simulink model "FOODSLIB"  (Simulink 4.00)
settings: Solver=ode5  SolverMode=SingleTasking  StartTime=0.0  StopTime=0  FixedStep=0  MaxStep=0  RelTol=1e-3  AbsTol=1e-6
undefined symbols (not defined in the file or in its folder): comptype, na, tref, turn
(part 2 of 2)

== system FOODSLIB/Unit  Operations/Single Stage Ultrafiltration/Advanced Transport Level (4) ==
  Hagen-Poiseuille  Model (1) : Subsystem
      settings: RTWFcnNameOpts=Auto  RTWFileNameOpts=Auto
  Mass Transfer (Film Theory) Model (2) : Subsystem
      settings: RTWFcnNameOpts=Auto  RTWFileNameOpts=Auto
  Model Selection : Constant  Value=1
  More Info : Subsystem
      settings: RTWFcnNameOpts=Auto  RTWFileNameOpts=Auto
      mask Display: disp('Help?')
  Mux1 : Mux  Inputs=4
      settings: DisplayOption=none
  Viscosity Model : Constant  Value=6
  out_1 : Outport  Port=1
  wires:
  Mux1/1 -> out_1/1
  Mass Transfer (Film Theory) Model (2)/1(out_1) -> Mux1/4
  Hagen-Poiseuille  Model (1)/1(out_1) -> Mux1/3
  Viscosity Model/1 -> Mux1/1
  Model Selection/1 -> Mux1/2

== system FOODSLIB/Unit  Operations/Single Stage Ultrafiltration/Basic Transport Level (3) ==
  Flux (L/h-m^2) : Constant  Value=17
  out_1 : Outport  Port=1
  wires:
  Flux (L/h-m^2)/1 -> out_1/1

== system FOODSLIB/Unit  Operations/Single Stage Ultrafiltration/Design ==
  Design Level : Constant  Value=4
  Economic Evaluation? : Constant  Value=turn('off')
  Microbial & Quality Assessment? : Constant  Value=turn('off')
  Mux2 : Mux  Inputs=3
      settings: DisplayOption=none
  out_1 : Outport  Port=1
  wires:
  Mux2/1 -> out_1/1
  Design Level/1 -> Mux2/1
  Microbial & Quality Assessment?/1 -> Mux2/2
  Economic Evaluation?/1 -> Mux2/3

== system FOODSLIB/Unit  Operations/Single Stage Ultrafiltration/Mass Balance Level (1) ==
  Ash Rejection Ratio : Constant  Value=[comptype('ash') 0.2]
  Carbohydrate Rejection Ratio : Constant  Value=[comptype('carbohydrate') 0]
  Component Fraction 10 Rejection Ratio : Constant  Value=[0 0]
  Component Fraction 7 Rejection Ratio : Constant  Value=[0 0]
  Component Fraction 8 Rejection Ratio : Constant  Value=[0 0]
  Component Fraction 9 Rejection Ratio : Constant  Value=[0 0]
  Fat Rejection Ratio : Constant  Value=[comptype('fat') 0]
  Fiber Rejection Ratio : Constant  Value=[comptype('fiber') 0]
  Mux : Mux  Inputs=10
      settings: DisplayOption=none
  Protein Rejection Ratio : Constant  Value=[comptype('protein') 0.9]
  Retentate Total Solids (w/w) : Constant  Value=0.2
  out_1 : Outport  Port=1
  wires:
  Fiber Rejection Ratio/1 -> Mux/4
  Carbohydrate Rejection Ratio/1 -> Mux/3
  Fat Rejection Ratio/1 -> Mux/5
  Protein Rejection Ratio/1 -> Mux/2
  Retentate Total Solids (w/w)/1 -> Mux/1
  Mux/1 -> out_1/1
  Ash Rejection Ratio/1 -> Mux/6
  Component Fraction 7 Rejection Ratio/1 -> Mux/7
  Component Fraction 8 Rejection Ratio/1 -> Mux/8
  Component Fraction 9 Rejection Ratio/1 -> Mux/9
  Component Fraction 10 Rejection Ratio/1 -> Mux/10

== system FOODSLIB/Unit  Operations/Single Stage Ultrafiltration/More Info ==
  note: Some Notes
  note: More Notes can go here

== system FOODSLIB/Unit  Operations/Single Stage Ultrafiltration/Ultrafiltration Cost Information ==
  Base Ultrafiltration Costing Model : Subsystem
      settings: RTWFcnNameOpts=Auto  RTWFileNameOpts=Auto
  Equipment Life (y) : Constant  Value=3
  Maintenance Labor (man-h/h operation) : Constant  Value=0.03
  Mux : Mux  Inputs=5
      settings: DisplayOption=none
  Operating Labor (man-h/h operation) : Constant  Value=1
  Salvage Value  (% of initial cost) : Constant  Value=0.1
  out_1 : Outport  Port=1
  wires:
  Maintenance Labor (man-h/h operation)/1 -> Mux/5
  Operating Labor (man-h/h operation)/1 -> Mux/4
  Equipment Life (y)/1 -> Mux/3
  Salvage Value  (% of initial cost)/1 -> Mux/2
  Base Ultrafiltration Costing Model/1(out_1) -> Mux/1
  Mux/1 -> out_1/1

== system FOODSLIB/Unit  Operations/Spray Dryer/Advanced Transport Level (4) ==
  Atomizer - Rotary  Vaned Wheel : Subsystem
      settings: RTWFcnNameOpts=Auto  RTWFileNameOpts=Auto
  Cone Angle (deg. from horizontal) : Constant  Value=60
  Critical  Moisture  Content (wb) : Constant  Value=0.25
  Cylindrical H:D Ratio : Constant  Value=1
  More Info : Subsystem
      settings: RTWFcnNameOpts=Auto  RTWFileNameOpts=Auto
      mask Display: disp('?')
  Mux1 : Mux  Inputs=6
      settings: DisplayOption=none
  Product Density (kg/m^3) : Constant  Value=605
  Viscosity Model : Constant  Value=1
  Out : Outport  Port=1
  wires:
  Mux1/1 -> Out/1
  Atomizer - Rotary  Vaned Wheel/1(out_1) -> Mux1/1
  Critical  Moisture  Content (wb)/1 -> Mux1/2
  Product Density (kg/m^3)/1 -> Mux1/3
  Cylindrical H:D Ratio/1 -> Mux1/4
  Cone Angle (deg. from horizontal)/1 -> Mux1/5
  Viscosity Model/1 -> Mux1/6

== system FOODSLIB/Unit  Operations/Spray Dryer/Design ==
  Design Level : Constant  Value=4
  Economic Evaluation? : Constant  Value=turn('off')
  Microbial & Quality Assessment? : Constant  Value=turn('off')
  Mux2 : Mux  Inputs=3
      settings: DisplayOption=none
  out_1 : Outport  Port=1
  wires:
  Mux2/1 -> out_1/1
  Design Level/1 -> Mux2/1
  Microbial & Quality Assessment?/1 -> Mux2/2
  Economic Evaluation?/1 -> Mux2/3

== system FOODSLIB/Unit  Operations/Spray Dryer/Energy Balance Level (2) ==
  Air Recycle Fraction : Constant  Value=0
  Dryer Air Inlet Temperature (C) : Constant  Value=170
  Dryer Air Outlet Temperature (C) : Constant  Value=90
  Dryer Heat Loss Rate (kJ/h) : Constant  Value=0.0
  Mux : Mux  Inputs=6
      settings: DisplayOption=none
  Operating Pressure (MPa) : Constant  Value=0.101325
  Product Temperature (C) : Constant  Value=75
  Outport : Outport  Port=1
  wires:
  Product Temperature (C)/1 -> Mux/1
  Dryer Air Inlet Temperature (C)/1 -> Mux/2
  Dryer Air Outlet Temperature (C)/1 -> Mux/3
  Mux/1 -> Outport/1
  Operating Pressure (MPa)/1 -> Mux/4
  Air Recycle Fraction/1 -> Mux/6
  Dryer Heat Loss Rate (kJ/h)/1 -> Mux/5

== system FOODSLIB/Unit  Operations/Spray Dryer/Mass Balance Level (1) ==
  Dry Product Total Solids (w/w) : Constant  Value=0.97
  out_1 : Outport  Port=1
  wires:
  Dry Product Total Solids (w/w)/1 -> out_1/1

== system FOODSLIB/Unit  Operations/Spray Dryer/Spray Dryer Cost Information ==
  Base Evaporator Costing Model : Subsystem
      settings: RTWFcnNameOpts=Auto  RTWFileNameOpts=Auto
  Equipment Life (y) : Constant  Value=10
  Maintenance Labor (man-h/h operation) : Constant  Value=0.06
  Mux : Mux  Inputs=5
      settings: DisplayOption=none
  Operating Labor (man-h/h operation) : Constant  Value=1
  Salvage Value  (% of initial cost) : Constant  Value=0.1
  out_1 : Outport  Port=1
  wires:
  Mux/1 -> out_1/1
  Base Evaporator Costing Model/1(out_1) -> Mux/1
  Salvage Value  (% of initial cost)/1 -> Mux/2
  Equipment Life (y)/1 -> Mux/3
  Operating Labor (man-h/h operation)/1 -> Mux/4
  Maintenance Labor (man-h/h operation)/1 -> Mux/5

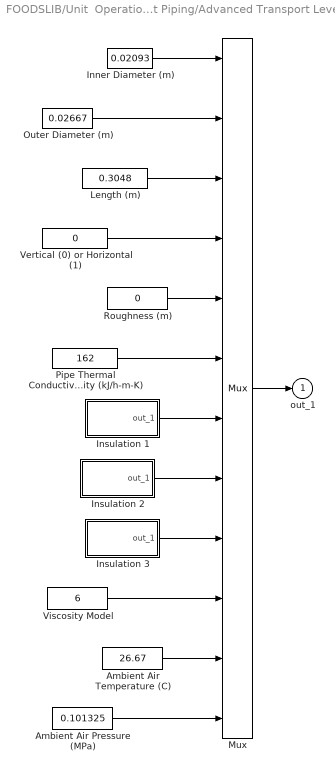
== system FOODSLIB/Unit  Operations/Straight Piping/Advanced Transport Level (4) ==
  Ambient Air Pressure (MPa) : Constant  Value=0.101325
  Ambient Air Temperature (C) : Constant  Value=26.67
  Inner Diameter (m) : Constant  Value=0.02093
  Insulation 1 : Subsystem
      settings: RTWFcnNameOpts=Auto  RTWFileNameOpts=Auto
  Insulation 2 : Subsystem
      settings: RTWFcnNameOpts=Auto  RTWFileNameOpts=Auto
  Insulation 3 : Subsystem
      settings: RTWFcnNameOpts=Auto  RTWFileNameOpts=Auto
  Length (m) : Constant  Value=0.3048
  Mux : Mux  Inputs=12
      settings: DisplayOption=none
  Outer Diameter (m) : Constant  Value=0.02667
  Pipe Thermal Conductivity (kJ/h-m-K) : Constant  Value=162
  Roughness (m) : Constant  Value=0
  Vertical (0) or Horizontal (1) : Constant  Value=0
  Viscosity Model : Constant  Value=6
  out_1 : Outport  Port=1
  wires:
  Inner Diameter (m)/1 -> Mux/1
  Outer Diameter (m)/1 -> Mux/2
  Length (m)/1 -> Mux/3
  Vertical (0) or Horizontal (1)/1 -> Mux/4
  Roughness (m)/1 -> Mux/5
  Pipe Thermal Conductivity (kJ/h-m-K)/1 -> Mux/6
  Insulation 1/1(out_1) -> Mux/7
  Insulation 2/1(out_1) -> Mux/8
  Insulation 3/1(out_1) -> Mux/9
  Mux/1 -> out_1/1
  Viscosity Model/1 -> Mux/10
  Ambient Air Temperature (C)/1 -> Mux/11
  Ambient Air Pressure (MPa)/1 -> Mux/12

== system FOODSLIB/Unit  Operations/Straight Piping/Design ==
  Design Level : Constant  Value=4
  Economic Evaluation? : Constant  Value=turn('off')
  Microbial & Quality Assessment? : Constant  Value=turn('off')
  Mux2 : Mux  Inputs=3
      settings: DisplayOption=none
  out_1 : Outport  Port=1
  wires:
  Mux2/1 -> out_1/1
  Design Level/1 -> Mux2/1
  Microbial & Quality Assessment?/1 -> Mux2/2
  Economic Evaluation?/1 -> Mux2/3

== system FOODSLIB/Unit  Operations/Straight Piping/Pipe Cost Information ==
  Base Evaporator Costing Model : Subsystem
      settings: RTWFcnNameOpts=Auto  RTWFileNameOpts=Auto
  Equipment Life (y) : Constant  Value=3
  Maintenance Labor (man-h/h operation) : Constant  Value=0.03
  Mux : Mux  Inputs=5
      settings: DisplayOption=none
  Operating Labor (man-h/h operation) : Constant  Value=1
  Salvage Value  (% of initial cost) : Constant  Value=0.1
  out_1 : Outport  Port=1
  wires:
  Maintenance Labor (man-h/h operation)/1 -> Mux/5
  Operating Labor (man-h/h operation)/1 -> Mux/4
  Equipment Life (y)/1 -> Mux/3
  Salvage Value  (% of initial cost)/1 -> Mux/2
  Base Evaporator Costing Model/1(out_1) -> Mux/1
  Mux/1 -> out_1/1

== system FOODSLIB/Unit  Operations/Sudden Expansion or Contraction/Advanced Transport Level (4) ==
  Diameter In (m) : Constant  Value=100
  Diameter Out (m) : Constant  Value=0.1023
  Equivalent Straight Pipe Roughness (m) : Constant  Value=0
  Mux : Mux  Inputs=4
      settings: DisplayOption=none
  Viscosity Model : Constant  Value=6
  out_1 : Outport  Port=1
  wires:
  Viscosity Model/1 -> Mux/4
  Equivalent Straight Pipe Roughness (m)/1 -> Mux/3
  Diameter Out (m)/1 -> Mux/2
  Diameter In (m)/1 -> Mux/1
  Mux/1 -> out_1/1

== system FOODSLIB/Unit  Operations/Sudden Expansion or Contraction/Design ==
  Design Level : Constant  Value=4
  Economic Evaluation? : Constant  Value=turn('off')
  Microbial & Quality Assessment? : Constant  Value=turn('off')
  Mux2 : Mux  Inputs=3
      settings: DisplayOption=none
  out_1 : Outport  Port=1
  wires:
  Economic Evaluation?/1 -> Mux2/3
  Microbial & Quality Assessment?/1 -> Mux2/2
  Design Level/1 -> Mux2/1
  Mux2/1 -> out_1/1

== system FOODSLIB/Unit  Operations/Sudden Expansion or Contraction/Fitting Cost Information ==
  Base Evaporator Costing Model : Subsystem
      settings: RTWFcnNameOpts=Auto  RTWFileNameOpts=Auto
  Equipment Life (y) : Constant  Value=3
  Maintenance Labor (man-h/h operation) : Constant  Value=0.03
  Mux : Mux  Inputs=5
      settings: DisplayOption=none
  Operating Labor (man-h/h operation) : Constant  Value=1
  Salvage Value  (% of initial cost) : Constant  Value=0.1
  out_1 : Outport  Port=1
  wires:
  Mux/1 -> out_1/1
  Base Evaporator Costing Model/1(out_1) -> Mux/1
  Salvage Value  (% of initial cost)/1 -> Mux/2
  Equipment Life (y)/1 -> Mux/3
  Operating Labor (man-h/h operation)/1 -> Mux/4
  Maintenance Labor (man-h/h operation)/1 -> Mux/5

== system FOODSLIB/Unit  Operations/Up To 6 Effect  Backward Feed  Evaporator/Advanced Transport Level (4) ==
  Evaporator Model Type (See ?) : Constant  Value=20
  Film Thickness (m) : Constant  Value=.0005
  Initial Guess at Number of Tubes : Constant  Value=35
  Minimum Average Fluid Velocity (m/s) : Constant  Value=2
  More Info : Subsystem
      settings: RTWFcnNameOpts=Auto  RTWFileNameOpts=Auto
      mask Display: disp('?')
  Mux1 : Mux  Inputs=8
      settings: DisplayOption=none
  Pipe Thermal Conductivity  (kJ/h-m-K) : Constant  Value=162
  Pipe Thickness (m) : Constant  Value=0.00391
  Tube Orientation: Horizontal (0); Vertical (1) : Constant  Value=1
  Viscosity Model For Product Side (See ?) : Constant  Value=1
  Out : Outport  Port=1
  wires:
  Mux1/1 -> Out/1
  Evaporator Model Type (See ?)/1 -> Mux1/1
  Tube Orientation: Horizontal (0); Vertical (1)/1 -> Mux1/2
  Viscosity Model For Product Side (See ?)/1 -> Mux1/3
  Pipe Thickness (m)/1 -> Mux1/4
  Pipe Thermal Conductivity  (kJ/h-m-K)/1 -> Mux1/5
  Minimum Average Fluid Velocity (m/s)/1 -> Mux1/6
  Film Thickness (m)/1 -> Mux1/7
  Initial Guess at Number of Tubes/1 -> Mux1/8

== system FOODSLIB/Unit  Operations/Up To 6 Effect  Backward Feed  Evaporator/Basic Transport Level (3) ==
  Effect 1: Overall Heat Transfer Coefficient (kJ/h-m^2-K) : Constant  Value=5400
  Effect 2: Overall Heat Transfer Coefficient (kJ/h-m^2-K) : Constant  Value=3600
  Effect 3: Overall Heat Transfer Coefficient (kJ/h-m^2-K) : Constant  Value=4090
  Effect 4: Overall Heat Transfer Coefficient (kJ/h-m^2-K) : Constant  Value=5400
  Effect 5: Overall Heat Transfer Coefficient (kJ/h-m^2-K) : Constant  Value=5400
  Effect 6: Overall Heat Transfer Coefficient (kJ/h-m^2-K) : Constant  Value=5400
  Inner Pipe Diameter (m) : Constant  Value=0.0525
  Mux1 : Mux  Inputs=8
      settings: DisplayOption=none
  Pipe Length (m) : Constant  Value=2.5
  out_1 : Outport  Port=1
  wires:
  Effect 5: Overall Heat Transfer Coefficient (kJ/h-m^2-K)/1 -> Mux1/5
  Pipe Length (m)/1 -> Mux1/8
  Inner Pipe Diameter (m)/1 -> Mux1/7
  Effect 4: Overall Heat Transfer Coefficient (kJ/h-m^2-K)/1 -> Mux1/4
  Effect 3: Overall Heat Transfer Coefficient (kJ/h-m^2-K)/1 -> Mux1/3
  Effect 2: Overall Heat Transfer Coefficient (kJ/h-m^2-K)/1 -> Mux1/2
  Effect 6: Overall Heat Transfer Coefficient (kJ/h-m^2-K)/1 -> Mux1/6
  Mux1/1 -> out_1/1
  Effect 1: Overall Heat Transfer Coefficient (kJ/h-m^2-K)/1 -> Mux1/1

== system FOODSLIB/Unit  Operations/Up To 6 Effect  Backward Feed  Evaporator/Design ==
  Design Level : Constant  Value=4
  Economic Evaluation? : Constant  Value=turn('off')
  Microbial & Quality Assessment? : Constant  Value=turn('off')
  Mux2 : Mux  Inputs=3
      settings: DisplayOption=none
  out_1 : Outport  Port=1
  wires:
  Mux2/1 -> out_1/1
  Design Level/1 -> Mux2/1
  Microbial & Quality Assessment?/1 -> Mux2/2
  Economic Evaluation?/1 -> Mux2/3

== system FOODSLIB/Unit  Operations/Up To 6 Effect  Backward Feed  Evaporator/Energy Balance Level (2) ==
  Boiling Point Rise Model : Constant  Value=3
  Exit Steam Quality : Constant  Value=0
  Last Effect Operating Pressure (MPa) : Constant  Value=0.007
  More Info : Subsystem
      settings: RTWFcnNameOpts=Auto  RTWFileNameOpts=Auto
      mask Display: disp('?')
  Mux : Mux  Inputs=3
      settings: DisplayOption=none
  out_1 : Outport  Port=1
  wires:
  Exit Steam Quality/1 -> Mux/2
  Last Effect Operating Pressure (MPa)/1 -> Mux/1
  Mux/1 -> out_1/1
  Boiling Point Rise Model/1 -> Mux/3

== system FOODSLIB/Unit  Operations/Up To 6 Effect  Backward Feed  Evaporator/Evaporator Cost Information ==
  Base Evaporator Costing Model : Subsystem
      settings: RTWFcnNameOpts=Auto  RTWFileNameOpts=Auto
  Equipment Life (y) : Constant  Value=10
  Maintenance Labor (man-h/h operation) : Constant  Value=0.015
  Mux : Mux  Inputs=5
      settings: DisplayOption=none
  Operating Labor (man-h/h operation) : Constant  Value=0.25
  Salvage Value  (% of initial cost) : Constant  Value=0.1
  out_1 : Outport  Port=1
  wires:
  Maintenance Labor (man-h/h operation)/1 -> Mux/5
  Operating Labor (man-h/h operation)/1 -> Mux/4
  Equipment Life (y)/1 -> Mux/3
  Salvage Value  (% of initial cost)/1 -> Mux/2
  Base Evaporator Costing Model/1(out_1) -> Mux/1
  Mux/1 -> out_1/1

== system FOODSLIB/Unit  Operations/Up To 6 Effect  Backward Feed  Evaporator/Mass Balance Level (1) ==
  Mux : Mux  Inputs=2
      settings: DisplayOption=none
  Number of Effects (Limited to 6) : Constant  Value=3
  Total Solids of Liquid Concentrate (w/w) : Constant  Value=0.48
  out_1 : Outport  Port=1
  wires:
  Total Solids of Liquid Concentrate (w/w)/1 -> Mux/2
  Number of Effects (Limited to 6)/1 -> Mux/1
  Mux/1 -> out_1/1

== system FOODSLIB/Unit  Operations/Up To 6 Effect  Forward Feed  Evaporator/Advanced Transport Level (4) ==
  Evaporator Model Type (See ?) : Constant  Value=20
  Film Thickness (m) : Constant  Value=.0005
  Initial Guess at Number of Tubes : Constant  Value=35
  Minimum Average Fluid Velocity (m/s) : Constant  Value=2
  More Info : Subsystem
      settings: RTWFcnNameOpts=Auto  RTWFileNameOpts=Auto
      mask Display: disp('?')
  Mux1 : Mux  Inputs=8
      settings: DisplayOption=none
  Pipe Thermal Conductivity  (kJ/h-m-K) : Constant  Value=162
  Pipe Thickness (m) : Constant  Value=0.00391
  Tube Orientation: Horizontal (0); Vertical (1) : Constant  Value=1
  Viscosity Model For Product Side (See ?) : Constant  Value=1
  Out : Outport  Port=1
  wires:
  Mux1/1 -> Out/1
  Evaporator Model Type (See ?)/1 -> Mux1/1
  Tube Orientation: Horizontal (0); Vertical (1)/1 -> Mux1/2
  Viscosity Model For Product Side (See ?)/1 -> Mux1/3
  Pipe Thickness (m)/1 -> Mux1/4
  Pipe Thermal Conductivity  (kJ/h-m-K)/1 -> Mux1/5
  Minimum Average Fluid Velocity (m/s)/1 -> Mux1/6
  Film Thickness (m)/1 -> Mux1/7
  Initial Guess at Number of Tubes/1 -> Mux1/8

== system FOODSLIB/Unit  Operations/Up To 6 Effect  Forward Feed  Evaporator/Basic Transport Level (3) ==
  Effect 1: Overall Heat Transfer Coefficient (kJ/h-m^2-K) : Constant  Value=5400
  Effect 2: Overall Heat Transfer Coefficient (kJ/h-m^2-K) : Constant  Value=3600
  Effect 3: Overall Heat Transfer Coefficient (kJ/h-m^2-K) : Constant  Value=4090
  Effect 4: Overall Heat Transfer Coefficient (kJ/h-m^2-K) : Constant  Value=5400
  Effect 5: Overall Heat Transfer Coefficient (kJ/h-m^2-K) : Constant  Value=5400
  Effect 6: Overall Heat Transfer Coefficient (kJ/h-m^2-K) : Constant  Value=5400
  Inner Pipe Diameter (m) : Constant  Value=0.0525
  Mux1 : Mux  Inputs=8
      settings: DisplayOption=none
  Pipe Length (m) : Constant  Value=2.5
  out_1 : Outport  Port=1
  wires:
  Effect 5: Overall Heat Transfer Coefficient (kJ/h-m^2-K)/1 -> Mux1/5
  Pipe Length (m)/1 -> Mux1/8
  Inner Pipe Diameter (m)/1 -> Mux1/7
  Effect 4: Overall Heat Transfer Coefficient (kJ/h-m^2-K)/1 -> Mux1/4
  Effect 3: Overall Heat Transfer Coefficient (kJ/h-m^2-K)/1 -> Mux1/3
  Effect 2: Overall Heat Transfer Coefficient (kJ/h-m^2-K)/1 -> Mux1/2
  Effect 6: Overall Heat Transfer Coefficient (kJ/h-m^2-K)/1 -> Mux1/6
  Mux1/1 -> out_1/1
  Effect 1: Overall Heat Transfer Coefficient (kJ/h-m^2-K)/1 -> Mux1/1

== system FOODSLIB/Unit  Operations/Up To 6 Effect  Forward Feed  Evaporator/Design ==
  Design Level : Constant  Value=4
  Economic Evaluation? : Constant  Value=turn('off')
  Microbial & Quality Assessment? : Constant  Value=turn('off')
  Mux2 : Mux  Inputs=3
      settings: DisplayOption=none
  out_1 : Outport  Port=1
  wires:
  Mux2/1 -> out_1/1
  Design Level/1 -> Mux2/1
  Microbial & Quality Assessment?/1 -> Mux2/2
  Economic Evaluation?/1 -> Mux2/3

== system FOODSLIB/Unit  Operations/Up To 6 Effect  Forward Feed  Evaporator/Energy Balance Level (2) ==
  Boiling Point Rise Model : Constant  Value=3
  Exit Steam Quality : Constant  Value=0
  Last Effect Operating Pressure (MPa) : Constant  Value=0.007
  More Info : Subsystem
      settings: RTWFcnNameOpts=Auto  RTWFileNameOpts=Auto
      mask Display: disp('?')
  Mux : Mux  Inputs=3
      settings: DisplayOption=none
  out_1 : Outport  Port=1
  wires:
  Exit Steam Quality/1 -> Mux/2
  Last Effect Operating Pressure (MPa)/1 -> Mux/1
  Mux/1 -> out_1/1
  Boiling Point Rise Model/1 -> Mux/3

== system FOODSLIB/Unit  Operations/Up To 6 Effect  Forward Feed  Evaporator/Evaporator Cost Information ==
  Base Evaporator Costing Model : Subsystem
      settings: RTWFcnNameOpts=Auto  RTWFileNameOpts=Auto
  Equipment Life (y) : Constant  Value=10
  Maintenance Labor (man-h/h operation) : Constant  Value=0.015
  Mux : Mux  Inputs=5
      settings: DisplayOption=none
  Operating Labor (man-h/h operation) : Constant  Value=0.25
  Salvage Value  (% of initial cost) : Constant  Value=0.1
  out_1 : Outport  Port=1
  wires:
  Maintenance Labor (man-h/h operation)/1 -> Mux/5
  Operating Labor (man-h/h operation)/1 -> Mux/4
  Equipment Life (y)/1 -> Mux/3
  Salvage Value  (% of initial cost)/1 -> Mux/2
  Base Evaporator Costing Model/1(out_1) -> Mux/1
  Mux/1 -> out_1/1

== system FOODSLIB/Unit  Operations/Up To 6 Effect  Forward Feed  Evaporator/Mass Balance Level (1) ==
  Mux : Mux  Inputs=2
      settings: DisplayOption=none
  Number of Effects (Limited to 6) : Constant  Value=3
  Total Solids of Liquid Concentrate (w/w) : Constant  Value=0.48
  out_1 : Outport  Port=1
  wires:
  Total Solids of Liquid Concentrate (w/w)/1 -> Mux/2
  Number of Effects (Limited to 6)/1 -> Mux/1
  Mux/1 -> out_1/1

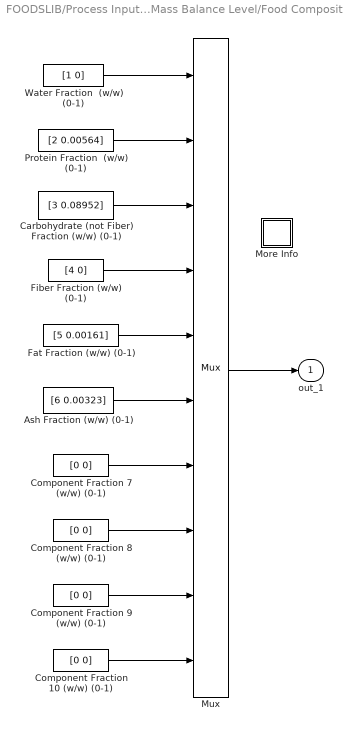
== system FOODSLIB/Process Inputs/Food/Mass Balance Level/Food Composition ==
  Ash Fraction (w/w) (0-1) : Constant  Value=[6 0.00323]
  Carbohydrate (not Fiber) Fraction (w/w) (0-1) : Constant  Value=[3 0.08952]
  Component Fraction 10 (w/w) (0-1) : Constant  Value=[0 0]
  Component Fraction 7 (w/w) (0-1) : Constant  Value=[0 0]
  Component Fraction 8 (w/w) (0-1) : Constant  Value=[0 0]
  Component Fraction 9 (w/w) (0-1) : Constant  Value=[0 0]
  Fat Fraction (w/w) (0-1) : Constant  Value=[5 0.00161]
  Fiber Fraction (w/w) (0-1) : Constant  Value=[4 0]
  More Info : Subsystem
      settings: RTWFcnNameOpts=Auto  RTWFileNameOpts=Auto
      mask Display: disp('?')
  Mux : Mux  Inputs=10
      settings: DisplayOption=none
  Protein Fraction  (w/w) (0-1) : Constant  Value=[2 0.00564]
  Water Fraction  (w/w) (0-1) : Constant  Value=[1 0]
  out_1 : Outport  Port=1
  wires:
  Mux/1 -> out_1/1
  Protein Fraction  (w/w) (0-1)/1 -> Mux/2
  Carbohydrate (not Fiber) Fraction (w/w) (0-1)/1 -> Mux/3
  Water Fraction  (w/w) (0-1)/1 -> Mux/1
  Fiber Fraction (w/w) (0-1)/1 -> Mux/4
  Fat Fraction (w/w) (0-1)/1 -> Mux/5
  Ash Fraction (w/w) (0-1)/1 -> Mux/6
  Component Fraction 7 (w/w) (0-1)/1 -> Mux/7
  Component Fraction 8 (w/w) (0-1)/1 -> Mux/8
  Component Fraction 9 (w/w) (0-1)/1 -> Mux/9
  Component Fraction 10 (w/w) (0-1)/1 -> Mux/10

== system FOODSLIB/Process Inputs/Steam Source/Economics Level/More Info ==
  note: Steam Source Costs are currently NOT set in this block.
      | Rather, they are set within ECONANAL.
      | (na = not available = 0)

== system FOODSLIB/Process Inputs/Steam Source/Energy Balance Level/More Info ==
  note: SUPER-HEATED STATE: Both the Temperature and Pressure must be set.
      | The Quality should be set to a value of 2.
  note: VAPOR-LIQUID STATE: Either the Temperature OR the Pressure may be set.
      | If both properties are set, the pressure will be used to determine the saturated
      | temperature. The saturated temperature will be used throughout the model.

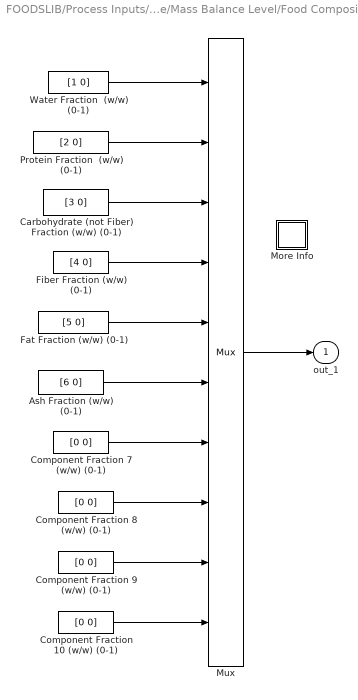
== system FOODSLIB/Process Inputs/Steam w/ known Mass Flowrate/Mass Balance Level/Food Composition ==
  Ash Fraction (w/w) (0-1) : Constant  Value=[6 0]
  Carbohydrate (not Fiber) Fraction (w/w) (0-1) : Constant  Value=[3 0]
  Component Fraction 10 (w/w) (0-1) : Constant  Value=[0 0]
  Component Fraction 7 (w/w) (0-1) : Constant  Value=[0 0]
  Component Fraction 8 (w/w) (0-1) : Constant  Value=[0 0]
  Component Fraction 9 (w/w) (0-1) : Constant  Value=[0 0]
  Fat Fraction (w/w) (0-1) : Constant  Value=[5 0]
  Fiber Fraction (w/w) (0-1) : Constant  Value=[4 0]
  More Info : Subsystem
      settings: RTWFcnNameOpts=Auto  RTWFileNameOpts=Auto
      mask Display: disp('?')
  Mux : Mux  Inputs=10
      settings: DisplayOption=none
  Protein Fraction  (w/w) (0-1) : Constant  Value=[2 0]
  Water Fraction  (w/w) (0-1) : Constant  Value=[1 0]
  out_1 : Outport  Port=1
  wires:
  Component Fraction 10 (w/w) (0-1)/1 -> Mux/10
  Component Fraction 9 (w/w) (0-1)/1 -> Mux/9
  Component Fraction 8 (w/w) (0-1)/1 -> Mux/8
  Component Fraction 7 (w/w) (0-1)/1 -> Mux/7
  Ash Fraction (w/w) (0-1)/1 -> Mux/6
  Fat Fraction (w/w) (0-1)/1 -> Mux/5
  Fiber Fraction (w/w) (0-1)/1 -> Mux/4
  Water Fraction  (w/w) (0-1)/1 -> Mux/1
  Carbohydrate (not Fiber) Fraction (w/w) (0-1)/1 -> Mux/3
  Protein Fraction  (w/w) (0-1)/1 -> Mux/2
  Mux/1 -> out_1/1

== system FOODSLIB/Process Inputs/Water Source/Economics Level/More Info ==
  note: Water Source Costs are currently NOT set in this block.
      | Rather, they are set within ECONANAL.
      | (na = not available = 0)

== system FOODSLIB/Process Inputs/Water Source/Energy Balance Level/More Info ==
  note: To specifiy a water source, the Quality must be set to zero.
  note: Only the Temperature may be set.

== system FOODSLIB/Unit  Operations/Heat Exchanger/Energy Balance Level (2)/More Info ==
  note: Flow Configuration:
      | Co-Current = 0
      | Counter-Current = 1

== system FOODSLIB/Unit  Operations/Heat Exchanger/Heat Exchanger Cost Information/Base Heat Exchanger Costing Model ==
  Base Cost ($) : Constant  Value=5500
  Base MSI : Constant  Value=300
  Base Size (m^2) : Constant  Value=13.9
  Maximum Size (m^2) : Constant  Value=18.6
  Minimim Size (m^2) : Constant  Value=9.3
  Mux : Mux  Inputs=6
      settings: DisplayOption=none
  Scaling Index : Constant  Value=0.65
  out_1 : Outport  Port=1
  wires:
  Maximum Size (m^2)/1 -> Mux/6
  Minimim Size (m^2)/1 -> Mux/5
  Scaling Index/1 -> Mux/4
  Base Cost ($)/1 -> Mux/3
  Base Size (m^2)/1 -> Mux/2
  Base MSI/1 -> Mux/1
  Mux/1 -> out_1/1

== system FOODSLIB/Unit  Operations/Holding Tube/Holding Tube Cost Information/Base Evaporator Costing Model ==
  Base Cost ($/m) : Constant  Value=164
  Base MSI : Constant  Value=904
  Base Size: Nominal Diameter (m) : Constant  Value=0.1016
  Maximum Size: Nominal Diameter (m) : Constant  Value=0.680
  Minimim Size:  Nominal Diameter (m) : Constant  Value=0.0178
  Mux : Mux  Inputs=6
      settings: DisplayOption=none
  Scaling Index : Constant  Value=0.973
  out_1 : Outport  Port=1
  wires:
  Mux/1 -> out_1/1
  Base MSI/1 -> Mux/1
  Base Size: Nominal Diameter (m)/1 -> Mux/2
  Base Cost ($/m)/1 -> Mux/3
  Scaling Index/1 -> Mux/4
  Minimim Size:  Nominal Diameter (m)/1 -> Mux/5
  Maximum Size: Nominal Diameter (m)/1 -> Mux/6

== system FOODSLIB/Unit  Operations/Mass Split/Evaporator Cost Information/Base Mass Split Costing Model ==
  Base Cost ($) : Constant  Value=110150
  Base MSI : Constant  Value=904
  Base Size : Constant  Value=1
  Maximum Size : Constant  Value=1
  Minimim Size : Constant  Value=1
  Mux : Mux  Inputs=6
      settings: DisplayOption=none
  Scaling Index : Constant  Value=0.54
  out_1 : Outport  Port=1
  wires:
  Maximum Size/1 -> Mux/6
  Minimim Size/1 -> Mux/5
  Scaling Index/1 -> Mux/4
  Base Cost ($)/1 -> Mux/3
  Base Size/1 -> Mux/2
  Base MSI/1 -> Mux/1
  Mux/1 -> out_1/1

== system FOODSLIB/Unit  Operations/Pipe Fitting/Fitting Cost Information/Base Evaporator Costing Model ==
  Base Cost ($) : Constant  Value=110150
  Base MSI : Constant  Value=904
  Base Size (m^2) : Constant  Value=100
  Maximum Size (m^2) : Constant  Value=740
  Minimim Size (m^2) : Constant  Value=9.3
  Mux : Mux  Inputs=6
      settings: DisplayOption=none
  Scaling Index : Constant  Value=0.54
  out_1 : Outport  Port=1
  wires:
  Mux/1 -> out_1/1
  Base MSI/1 -> Mux/1
  Base Size (m^2)/1 -> Mux/2
  Base Cost ($)/1 -> Mux/3
  Scaling Index/1 -> Mux/4
  Minimim Size (m^2)/1 -> Mux/5
  Maximum Size (m^2)/1 -> Mux/6

== system FOODSLIB/Unit  Operations/Point Mix/Point Mix Cost Information/Base Mass Split Costing Model ==
  Base Cost ($) : Constant  Value=110150
  Base MSI : Constant  Value=904
  Base Size : Constant  Value=1
  Maximum Size : Constant  Value=1
  Minimim Size : Constant  Value=1
  Mux : Mux  Inputs=6
      settings: DisplayOption=none
  Scaling Index : Constant  Value=0.54
  out_1 : Outport  Port=1
  wires:
  Maximum Size/1 -> Mux/6
  Minimim Size/1 -> Mux/5
  Scaling Index/1 -> Mux/4
  Base Cost ($)/1 -> Mux/3
  Base Size/1 -> Mux/2
  Base MSI/1 -> Mux/1
  Mux/1 -> out_1/1

== system FOODSLIB/Unit  Operations/Point Mix 3/Point Mix Cost Information/Base Mass Split Costing Model ==
  Base Cost ($) : Constant  Value=110150
  Base MSI : Constant  Value=904
  Base Size : Constant  Value=1
  Maximum Size : Constant  Value=1
  Minimim Size : Constant  Value=1
  Mux : Mux  Inputs=6
      settings: DisplayOption=none
  Scaling Index : Constant  Value=0.54
  out_1 : Outport  Port=1
  wires:
  Mux/1 -> out_1/1
  Base MSI/1 -> Mux/1
  Base Size/1 -> Mux/2
  Base Cost ($)/1 -> Mux/3
  Scaling Index/1 -> Mux/4
  Minimim Size/1 -> Mux/5
  Maximum Size/1 -> Mux/6

== system FOODSLIB/Unit  Operations/Pump/Pump Cost Information/Base Evaporator Costing Model ==
  Base Cost ($) : Constant  Value=110150
  Base MSI : Constant  Value=904
  Base Size: Nominal Diameter (m) : Constant  Value=0.0254
  Maximum Size: Nominal Diameter (m) : Constant  Value=0.03
  Minimim Size:  Nominal Diameter (m) : Constant  Value=0.01
  Mux : Mux  Inputs=6
      settings: DisplayOption=none
  Scaling Index : Constant  Value=0.54
  out_1 : Outport  Port=1
  wires:
  Mux/1 -> out_1/1
  Base MSI/1 -> Mux/1
  Base Size: Nominal Diameter (m)/1 -> Mux/2
  Base Cost ($)/1 -> Mux/3
  Scaling Index/1 -> Mux/4
  Minimim Size:  Nominal Diameter (m)/1 -> Mux/5
  Maximum Size: Nominal Diameter (m)/1 -> Mux/6

== system FOODSLIB/Unit  Operations/Single Effect Evaporator/Advanced Transport Level (4)/More Info ==
  note: Evaporator Model Types currently include:
      | Vertical-tube recirulating evaporator - natural circulation = 1
      | Vertical-tube recirculation evaporator - forced circulation = 2

== system FOODSLIB/Unit  Operations/Single Effect Evaporator/Energy Balance Level (2)/More Info ==
  note: Boiling Point Rise Models currently include:
      | None = 0
      | Molecular Concentration = 1
      | Sugar Solutions = 2

== system FOODSLIB/Unit  Operations/Single Effect Evaporator/Evaporator Cost Information/Base Evaporator Costing Model ==
  Base Cost ($) : Constant  Value=23000
  Base MSI : Constant  Value=300
  Base Size (m^2) : Constant  Value=92.9
  Maximum Size (m^2) : Constant  Value=9290.3
  Minimim Size (m^2) : Constant  Value=0.93
  Mux : Mux  Inputs=6
      settings: DisplayOption=none
  Scaling Index : Constant  Value=0.68
  out_1 : Outport  Port=1
  wires:
  Mux/1 -> out_1/1
  Maximum Size (m^2)/1 -> Mux/6
  Minimim Size (m^2)/1 -> Mux/5
  Scaling Index/1 -> Mux/4
  Base Cost ($)/1 -> Mux/3
  Base Size (m^2)/1 -> Mux/2
  Base MSI/1 -> Mux/1

== system FOODSLIB/Unit  Operations/Single Stage Ultrafiltration/Advanced Transport Level (4)/Hagen-Poiseuille  Model (1) ==
  Mean Pore Diameter (microns) : Constant  Value=0.0175
  Mux : Mux  Inputs=4
      settings: DisplayOption=none
  Pore Density (pores/cm^2) : Constant  Value=3e9
  Skin thickness (microns) : Constant  Value=0.2
  Transmembrane Pressure (MPa) : Constant  Value=0.1
  out_1 : Outport  Port=1
  wires:
  Pore Density (pores/cm^2)/1 -> Mux/4
  Skin thickness (microns)/1 -> Mux/3
  Mean Pore Diameter (microns)/1 -> Mux/2
  Transmembrane Pressure (MPa)/1 -> Mux/1
  Mux/1 -> out_1/1

== system FOODSLIB/Unit  Operations/Single Stage Ultrafiltration/Advanced Transport Level (4)/Mass Transfer (Film Theory) Model (2) ==
  Diffusivity (cm^2/s) : Constant  Value=7e-7
  Gel layer concentration (w/w) : Constant  Value=0.22
  Hydraulic (tube/fiber) Diameter (m) : Constant  Value=0.0011
  Model Constants : Subsystem
      settings: RTWFcnNameOpts=Auto  RTWFileNameOpts=Auto
  Mux : Mux  Inputs=6
      settings: DisplayOption=none
  Number of tubes/fibers : Constant  Value=660
  Tube/Fiber Length (m) : Constant  Value=0.635
  out_1 : Outport  Port=1
  wires:
  Gel layer concentration (w/w)/1 -> Mux/5
  Model Constants/1(out_1) -> Mux/6
  Diffusivity (cm^2/s)/1 -> Mux/4
  Number of tubes/fibers/1 -> Mux/3
  Tube/Fiber Length (m)/1 -> Mux/2
  Hydraulic (tube/fiber) Diameter (m)/1 -> Mux/1
  Mux/1 -> out_1/1

== system FOODSLIB/Unit  Operations/Single Stage Ultrafiltration/Advanced Transport Level (4)/More Info ==
  note: Evaporator Model Types currently include:
      | Vertical-tube recirulating evaporator - natural circulation = 1
      | Vertical-tube recirculation evaporator - forced circulation = 2

== system FOODSLIB/Unit  Operations/Single Stage Ultrafiltration/Ultrafiltration Cost Information/Base Ultrafiltration Costing Model ==
  Base Cost ($) : Constant  Value=110150
  Base MSI : Constant  Value=904
  Base Size (m^2) : Constant  Value=100
  Maximum Size (m^2) : Constant  Value=740
  Minimim Size (m^2) : Constant  Value=9.3
  Mux : Mux  Inputs=6
      settings: DisplayOption=none
  Scaling Index : Constant  Value=0.54
  out_1 : Outport  Port=1
  wires:
  Maximum Size (m^2)/1 -> Mux/6
  Minimim Size (m^2)/1 -> Mux/5
  Scaling Index/1 -> Mux/4
  Base Cost ($)/1 -> Mux/3
  Base Size (m^2)/1 -> Mux/2
  Base MSI/1 -> Mux/1
  Mux/1 -> out_1/1

== system FOODSLIB/Unit  Operations/Spray Dryer/Advanced Transport Level (4)/Atomizer - Rotary  Vaned Wheel ==
  "Mean Droplet Diameter (m) {Value overrides calculated value}" : Constant  Value=0
  Mux : Mux  Inputs=5
      settings: DisplayOption=none
  Number of Vanes : Constant  Value=36
  Vane Height (m) : Constant  Value=0.03
  Wheel Diameter (m) : Constant  Value=0.25
  Wheel Speed (rpm) : Constant  Value=12000
  out_1 : Outport  Port=1
  wires:
  Vane Height (m)/1 -> Mux/5
  Number of Vanes/1 -> Mux/4
  Wheel Diameter (m)/1 -> Mux/3
  Wheel Speed (rpm)/1 -> Mux/2
  "Mean Droplet Diameter (m) {Value overrides calculated value}"/1 -> Mux/1
  Mux/1 -> out_1/1

== system FOODSLIB/Unit  Operations/Spray Dryer/Advanced Transport Level (4)/More Info ==
  note: Evaporator Model Types currently include:
      | Vertical-tube recirulating evaporator - natural circulation = 1
      | Vertical-tube recirculation evaporator - forced circulation = 2

== system FOODSLIB/Unit  Operations/Spray Dryer/Spray Dryer Cost Information/Base Evaporator Costing Model ==
  Base Cost ($) : Constant  Value=150000
  Base MSI : Constant  Value=300
  Base Size (kg water/h) : Constant  Value=2268.
  Maximum Size (kg water/h) : Constant  Value=9071.8
  Minimim Size (kg water/h) : Constant  Value=113.4
  Mux : Mux  Inputs=6
      settings: DisplayOption=none
  Scaling Index : Constant  Value=0.71
  out_1 : Outport  Port=1
  wires:
  Mux/1 -> out_1/1
  Base MSI/1 -> Mux/1
  Base Size (kg water/h)/1 -> Mux/2
  Base Cost ($)/1 -> Mux/3
  Scaling Index/1 -> Mux/4
  Minimim Size (kg water/h)/1 -> Mux/5
  Maximum Size (kg water/h)/1 -> Mux/6

== system FOODSLIB/Unit  Operations/Straight Piping/Advanced Transport Level (4)/Insulation 1 ==
  Mux1 : Mux  Inputs=2
      settings: DisplayOption=none
  Thermal Conductivity (kJ/h-m-K) : Constant  Value=0.2304
  Thickness (m) : Constant  Value=0.0381
  out_1 : Outport  Port=1
  wires:
  Mux1/1 -> out_1/1
  Thickness (m)/1 -> Mux1/1
  Thermal Conductivity (kJ/h-m-K)/1 -> Mux1/2

== system FOODSLIB/Unit  Operations/Straight Piping/Advanced Transport Level (4)/Insulation 2 ==
  Mux1 : Mux  Inputs=2
      settings: DisplayOption=none
  Thermal Conductivity (kJ/h-m-K) : Constant  Value=0.0
  Thickness (m) : Constant  Value=0.0
  out_1 : Outport  Port=1
  wires:
  Mux1/1 -> out_1/1
  Thickness (m)/1 -> Mux1/1
  Thermal Conductivity (kJ/h-m-K)/1 -> Mux1/2

== system FOODSLIB/Unit  Operations/Straight Piping/Advanced Transport Level (4)/Insulation 3 ==
  Mux1 : Mux  Inputs=2
      settings: DisplayOption=none
  Thermal Conductivity (kJ/h-m-K) : Constant  Value=0.0
  Thickness (m) : Constant  Value=0
  out_1 : Outport  Port=1
  wires:
  Mux1/1 -> out_1/1
  Thickness (m)/1 -> Mux1/1
  Thermal Conductivity (kJ/h-m-K)/1 -> Mux1/2

== system FOODSLIB/Unit  Operations/Straight Piping/Pipe Cost Information/Base Evaporator Costing Model ==
  Base Cost ($) : Constant  Value=110150
  Base MSI : Constant  Value=904
  Base Size: Nominal Diameter (m) : Constant  Value=0.0254
  Maximum Size: Nominal Diameter (m) : Constant  Value=0.03
  Minimim Size:  Nominal Diameter (m) : Constant  Value=0.01
  Mux : Mux  Inputs=6
      settings: DisplayOption=none
  Scaling Index : Constant  Value=0.54
  out_1 : Outport  Port=1
  wires:
  Maximum Size: Nominal Diameter (m)/1 -> Mux/6
  Minimim Size:  Nominal Diameter (m)/1 -> Mux/5
  Scaling Index/1 -> Mux/4
  Base Cost ($)/1 -> Mux/3
  Base Size: Nominal Diameter (m)/1 -> Mux/2
  Base MSI/1 -> Mux/1
  Mux/1 -> out_1/1

== system FOODSLIB/Unit  Operations/Sudden Expansion or Contraction/Fitting Cost Information/Base Evaporator Costing Model ==
  Base Cost ($) : Constant  Value=110150
  Base MSI : Constant  Value=904
  Base Size (m^2) : Constant  Value=100
  Maximum Size (m^2) : Constant  Value=740
  Minimim Size (m^2) : Constant  Value=9.3
  Mux : Mux  Inputs=6
      settings: DisplayOption=none
  Scaling Index : Constant  Value=0.54
  out_1 : Outport  Port=1
  wires:
  Mux/1 -> out_1/1
  Base MSI/1 -> Mux/1
  Base Size (m^2)/1 -> Mux/2
  Base Cost ($)/1 -> Mux/3
  Scaling Index/1 -> Mux/4
  Minimim Size (m^2)/1 -> Mux/5
  Maximum Size (m^2)/1 -> Mux/6

== system FOODSLIB/Unit  Operations/Up To 6 Effect  Backward Feed  Evaporator/Advanced Transport Level (4)/More Info ==
  note: Evaporator Model Types currently include:
      | Vertical-tube recirulating evaporator - natural circulation = 1
      | Vertical-tube recirculation evaporator - forced circulation = 2

== system FOODSLIB/Unit  Operations/Up To 6 Effect  Backward Feed  Evaporator/Energy Balance Level (2)/More Info ==
  note: Boiling Point Rise Models currently include:
      | None = 0
      | Molecular Concentration = 1
      | Sugar Solutions = 2

== system FOODSLIB/Unit  Operations/Up To 6 Effect  Backward Feed  Evaporator/Evaporator Cost Information/Base Evaporator Costing Model ==
  Base Cost ($) : Constant  Value=23000
  Base MSI : Constant  Value=300
  Base Size (m^2) : Constant  Value=92.9
  Maximum Size (m^2) : Constant  Value=9290.3
  Minimim Size (m^2) : Constant  Value=0.93
  Mux : Mux  Inputs=6
      settings: DisplayOption=none
  Scaling Index : Constant  Value=0.68
  out_1 : Outport  Port=1
  wires:
  Maximum Size (m^2)/1 -> Mux/6
  Minimim Size (m^2)/1 -> Mux/5
  Scaling Index/1 -> Mux/4
  Base Cost ($)/1 -> Mux/3
  Base Size (m^2)/1 -> Mux/2
  Base MSI/1 -> Mux/1
  Mux/1 -> out_1/1

== system FOODSLIB/Unit  Operations/Up To 6 Effect  Forward Feed  Evaporator/Advanced Transport Level (4)/More Info ==
  note: Evaporator Model Types currently include:
      | Vertical-tube recirulating evaporator - natural circulation = 1
      | Vertical-tube recirculation evaporator - forced circulation = 2

== system FOODSLIB/Unit  Operations/Up To 6 Effect  Forward Feed  Evaporator/Energy Balance Level (2)/More Info ==
  note: Boiling Point Rise Models currently include:
      | None = 0
      | Molecular Concentration = 1
      | Sugar Solutions = 2

== system FOODSLIB/Unit  Operations/Up To 6 Effect  Forward Feed  Evaporator/Evaporator Cost Information/Base Evaporator Costing Model ==
  Base Cost ($) : Constant  Value=23000
  Base MSI : Constant  Value=300
  Base Size (m^2) : Constant  Value=92.9
  Maximum Size (m^2) : Constant  Value=9290.3
  Minimim Size (m^2) : Constant  Value=0.93
  Mux : Mux  Inputs=6
      settings: DisplayOption=none
  Scaling Index : Constant  Value=0.68
  out_1 : Outport  Port=1
  wires:
  Maximum Size (m^2)/1 -> Mux/6
  Minimim Size (m^2)/1 -> Mux/5
  Scaling Index/1 -> Mux/4
  Base Cost ($)/1 -> Mux/3
  Base Size (m^2)/1 -> Mux/2
  Base MSI/1 -> Mux/1
  Mux/1 -> out_1/1

== system FOODSLIB/Process Inputs/Food/Mass Balance Level/Food Composition/More Info ==
  note: Food Stream Compositions may be specified with up to 10 components.
      | The first component must ALWAYS be water.
  note: A check is made by the S-function feeds.m to ensure that the mass fractions
      | sum to 1. In the event that the sum of the mass fractions is less than 1,
      | the watermass fraction is recalculated to bring the sum up to 1.
  note: Each component is described by two values: type and mass fraction.
      | The values must be entered as [type mass_fraction] in the Constant Block.
      |
      | Example: A protein concentration of 4% (w/w) is entered as [2 0.04]
  note: Currently recognized component types are:
      | water =1
      | protein = 2
      | carbohydrate (not fiber) = 3
      | fiber = 4
      | fat = 5
      | ash = 6

== system FOODSLIB/Process Inputs/Steam w/ known Mass Flowrate/Mass Balance Level/Food Composition/More Info ==
  note: Currently recognized component types are:
      | water =1
      | protein = 2
      | carbohydrate (not fiber) = 3
      | fiber = 4
      | fat = 5
      | ash = 6
  note: Each component is described by two values: type and mass fraction.
      | The values must be entered as [type mass_fraction] in the Constant Block.
  note: A check is made by feeds.m to ensure that the mass fractions sum to 1.
      | In the event that the sum of the mass fractions is less than 1, the water
      | mass fraction is recalculated to bring the sum up to 1.
  note: Food Stream Compositions may be specified with up to 10 components.
      | The first component must ALWAYS be water.

== system FOODSLIB/Unit  Operations/Single Stage Ultrafiltration/Advanced Transport Level (4)/Mass Transfer (Film Theory) Model (2)/Model Constants ==
  A Coefficient : Constant  Value=0.2
  Alpha Exponent : Constant  Value=0.47
  Beta Exponent : Constant  Value=0.33
  Default to Leveque or  Colburn-Chilton Models : Constant  Value=1
  Mux : Mux  Inputs=5
      settings: DisplayOption=none
  w Exponent : Constant  Value=0
  out_1 : Outport  Port=1
  wires:
  Mux/1 -> out_1/1
  Default to Leveque or  Colburn-Chilton Models/1 -> Mux/1
  A Coefficient/1 -> Mux/2
  Alpha Exponent/1 -> Mux/3
  Beta Exponent/1 -> Mux/4
  w Exponent/1 -> Mux/5
